simulink model "simulink_mecha"  (R2016b)
settings: Solver=VariableStepAuto  StartTime=0.0  StopTime=50  RelTol=1e-3
libraries: aerolibutil x1, simulink x1
settings Model: Creator=Utente  LastModifiedBy=liana

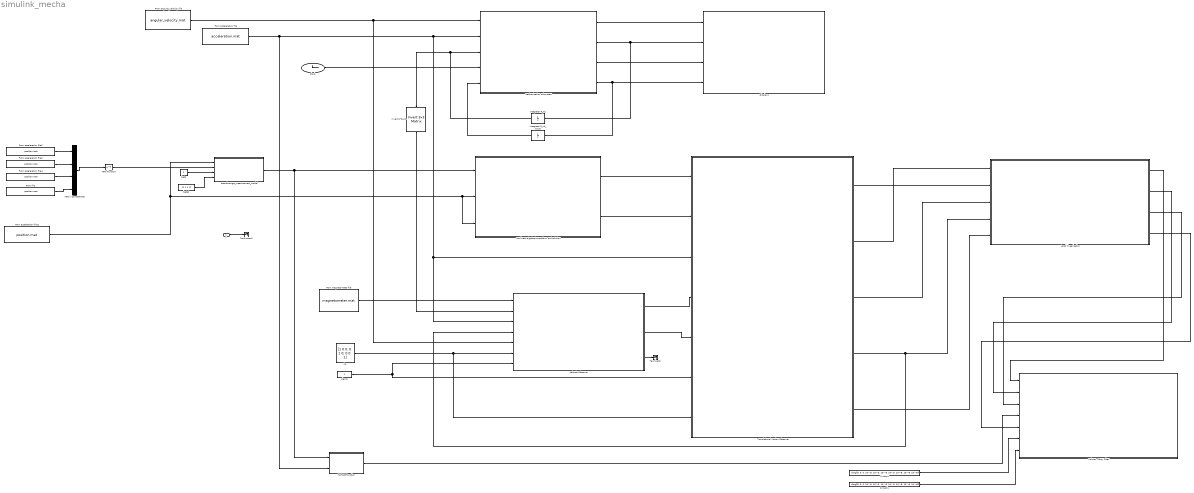
== system simulink_mecha ==
  f : Inport
  Attitude Observer : Subsystem
  Clock : Clock
  Displays : Subsystem
  From acceleration file : FromFile  FileName=acceleration.mat  SampleTime=0
  From acceleration file{1..4} (4 alike) : FromFile  FileName=position.mat  SampleTime=0
  From angular_velocity file : FromFile  FileName=angular_velocity.mat  SampleTime=0
  From file : FromFile  FileName=position.mat  SampleTime=0
  From magnetometer file : FromFile  FileName=magnetometer.mat  SampleTime=0  InterpolationWithinTimeRange=Zero order hold
  Integrator R_nb : Integrator
  Integrator R_nb_noise : Integrator
  Invert of R_nb : aerolibutil/Invert  3x3 Matrix
  Kalman - Bucy Filter : Subsystem
  Kp : Constant  Value=[1 0 0; 0 1 0; 0 0 1]
  Local linearization : Subsystem
  MATLAB Function : MATLAB Function  TreatAsAtomicUnit=on
  Math Function : Math  Operator=transpose  SaturateOnIntegerOverflow=on
  Matrix Concatenate : Concatenate  NumInputs=4  Mode=Multidimensional array  ConcatenateDimension=2
  Mechanisation subsystem : Subsystem
  Nonlinear algebraic transform and solution : Subsystem
  Q matrix : Constant  Value=diag([0, 0, 0, 10^-5, 10^-3, 10^-3, 10^-3, 10^-8, 10^-8, 10^-8])
  R matrix : Constant  Value=diag([0, 0, 0, 10^-5, 10^-3, 10^-3, 10^-3, 10^-8, 10^-8, 10^-8])
  Terminator : Terminator
  Terminator1 : Terminator
  Translational Motion Observer : Subsystem
  beta : Constant
  beta1 : Constant  Value=[1 1 1 1]
  pseudorange_measurement_model : MATLAB Function  TreatAsAtomicUnit=on
  sigma : Constant
  wires:
  From angular_velocity file/1 -> Attitude Observer/5(w_ib), Mechanisation subsystem/1(w_ib)
  Clock/1 -> Mechanisation subsystem/4(t)
  Mechanisation subsystem/2(R_nb_dot) -> Integrator R_nb/1, Displays/2(R_nb_dot)
  Integrator R_nb/1 -> Invert of R_nb/1, Mechanisation subsystem/3(R_nb)
  Mechanisation subsystem/1(v_n_dot) -> Displays/1(v_n_dot)
  Mechanisation subsystem/3(v_n_dot_noise) -> Displays/3(v_n_dot_noise)
  Mechanisation subsystem/4(R_nb_dot_noise) -> Integrator R_nb_noise/1, Displays/4(R_nb_dot_noise)
  Integrator R_nb_noise/1 -> Mechanisation subsystem/5(R_nb_noise)
  Invert of R_nb/1 -> Attitude Observer/2(R_bn)
  From magnetometer file/1 -> Attitude Observer/1(m_b_mag)
  Nonlinear algebraic transform and solution/1(delta) -> Translational Motion Observer/1(delta)
  Translational Motion Observer/4(f_n_stim) -> Local linearization/4(f_n_stim), Attitude Observer/4(f_n_stim)
  Attitude Observer/1(J) -> Translational Motion Observer/4(J)
  Attitude Observer/2(R_nb_stim) -> Translational Motion Observer/5(R_nb_stim)
  Attitude Observer/3(b_stim) -> Terminator/1
  From acceleration file1/1 -> pseudorange_measurement_model/1(p_n), Nonlinear algebraic transform and solution/3(p0), Nonlinear algebraic transform and solution/2(p)
  Kp/1 -> Translational Motion Observer/7(Kp), Attitude Observer/6(Kp)
  sigma/1 -> Translational Motion Observer/6(sigma), Attitude Observer/7(sigma)
  Translational Motion Observer/2(p_n_stim) -> Local linearization/1(p_n_stim)
  Translational Motion Observer/3(v_n_stim) -> Local linearization/3(v_n_stim)
  Nonlinear algebraic transform and solution/2(C_dx) -> Translational Motion Observer/2(C_dx)
  Translational Motion Observer/5(system) -> Local linearization/5(system)
  Translational Motion Observer/1(beta_stim) -> Local linearization/2(beta_stim)
  Local linearization/1(AL) -> Kalman - Bucy Filter/1(AL)
  Local linearization/2(BL) -> Kalman - Bucy Filter/2(BL)
  Local linearization/3(CL) -> Kalman - Bucy Filter/3(CL)
  MATLAB Function/1(z_k) -> Kalman - Bucy Filter/4(sensors measurements)
  From acceleration file/1 -> MATLAB Function/2(f_n), Attitude Observer/3(f_b), Translational Motion Observer/3(f_b_imu), Mechanisation subsystem/2(f_b)
  pseudorange_measurement_model/1(y) -> MATLAB Function/1(range), Nonlinear algebraic transform and solution/1(y)
  Local linearization/4(U) -> Kalman - Bucy Filter/5(U)
  f/1 -> Terminator1/1
  beta/1 -> pseudorange_measurement_model/3(beta)
  beta1/1 -> pseudorange_measurement_model/4(epsilon)
  From acceleration file2/1 -> Matrix Concatenate/1
  From acceleration file3/1 -> Matrix Concatenate/2
  From acceleration file4/1 -> Matrix Concatenate/3
  From file/1 -> Matrix Concatenate/4
  Matrix Concatenate/1 -> Math Function/1
  Math Function/1 -> pseudorange_measurement_model/2(p_n_i)
  R matrix/1 -> Kalman - Bucy Filter/6(R)
  Q matrix/1 -> Kalman - Bucy Filter/7(Q)

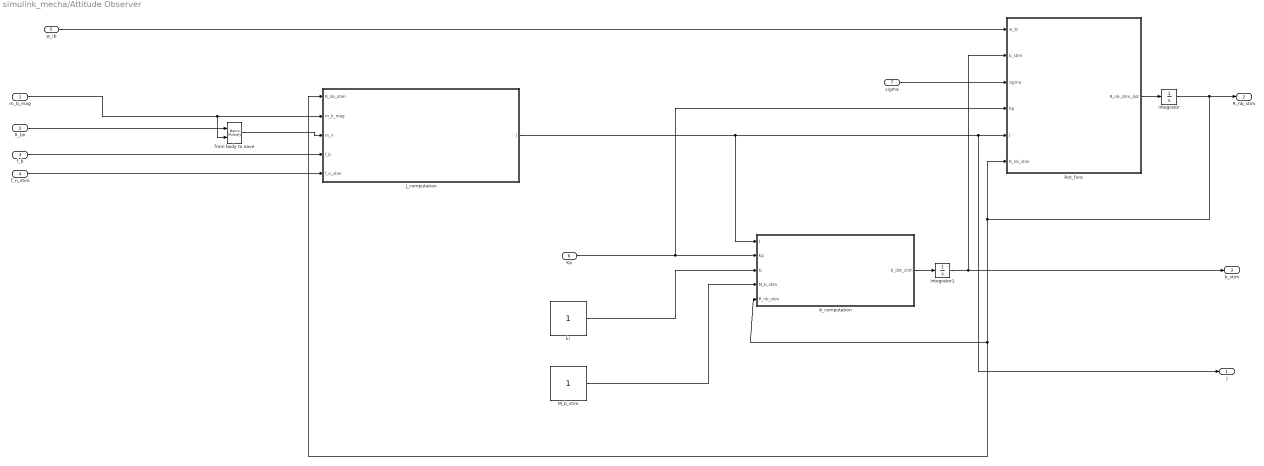
== system simulink_mecha/Attitude Observer ==
  m_b_mag : Inport
  R_bn : Inport  Port=2
  f_b : Inport  Port=3
  f_n_stim : Inport  Port=4
  w_ib : Inport  Port=5
  Kp : Inport  Port=6
  sigma : Inport  Port=7
  Integrator : Integrator
  Integrator1 : Integrator
  J_computation : Subsystem
  M_b_stim : Constant
  Rot_func : MATLAB Function  TreatAsAtomicUnit=on
  b_computation : MATLAB Function  TreatAsAtomicUnit=on
  from body to nave : Product  Multiplication=Matrix(*)
  ki : Constant
  J : Outport
  R_nb_stim : Outport  Port=2
  b_stim : Outport  Port=3
  wires:
  m_b_mag/1 -> from body to nave/2, J_computation/2(m_b_mag)
  Rot_func/1(R_nb_stim_dot) -> Integrator/1
  b_computation/1(b_dot_stim) -> Integrator1/1
  Integrator/1 -> J_computation/1(R_nb_stim), b_computation/5(R_nb_stim), Rot_func/6(R_nb_stim), R_nb_stim/1
  Integrator1/1 -> b_stim/1, Rot_func/2(b_stim)
  from body to nave/1 -> J_computation/3(m_n)
  f_b/1 -> J_computation/4(f_b)
  f_n_stim/1 -> J_computation/5(f_n_stim)
  J_computation/1(J) -> b_computation/1(J), J/1, Rot_func/5(J)
  Kp/1 -> Rot_func/4(Kp), b_computation/2(Kp)
  ki/1 -> b_computation/3(ki)
  M_b_stim/1 -> b_computation/4(M_b_stim)
  sigma/1 -> Rot_func/3(sigma)
  w_ib/1 -> Rot_func/1(w_ib)
  R_bn/1 -> from body to nave/1

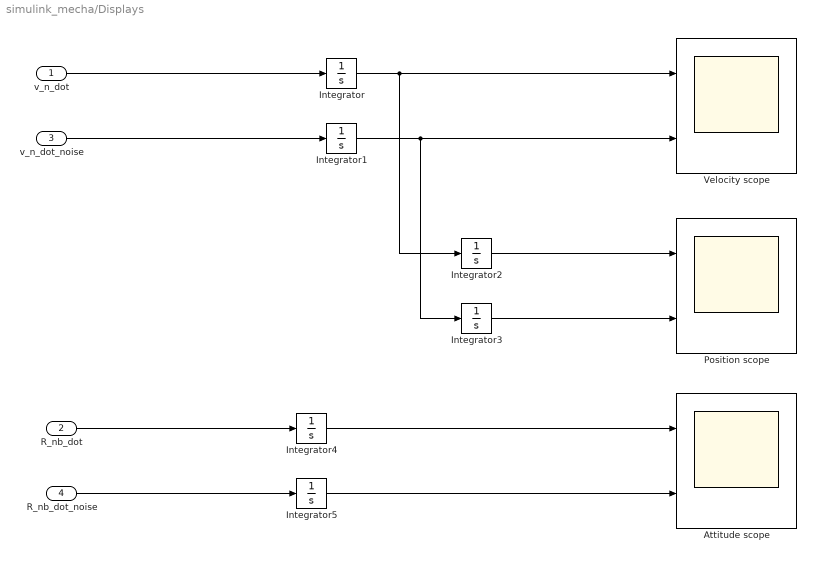
== system simulink_mecha/Displays ==
  v_n_dot : Inport
  R_nb_dot : Inport  Port=2
  v_n_dot_noise : Inport  Port=3
  R_nb_dot_noise : Inport  Port=4
  Attitude scope : Scope  NumInputPorts=2
  Integrator{,1..5} (6 alike) : Integrator
  Position scope : Scope  NumInputPorts=2
  Velocity scope : Scope  NumInputPorts=2
  wires:
  v_n_dot/1 -> Integrator/1
  v_n_dot_noise/1 -> Integrator1/1
  Integrator/1 -> Integrator2/1, Velocity scope/1
  Integrator1/1 -> Integrator3/1, Velocity scope/2
  Integrator2/1 -> Position scope/1
  Integrator3/1 -> Position scope/2
  R_nb_dot/1 -> Integrator4/1
  R_nb_dot_noise/1 -> Integrator5/1
  Integrator4/1 -> Attitude scope/1
  Integrator5/1 -> Attitude scope/2

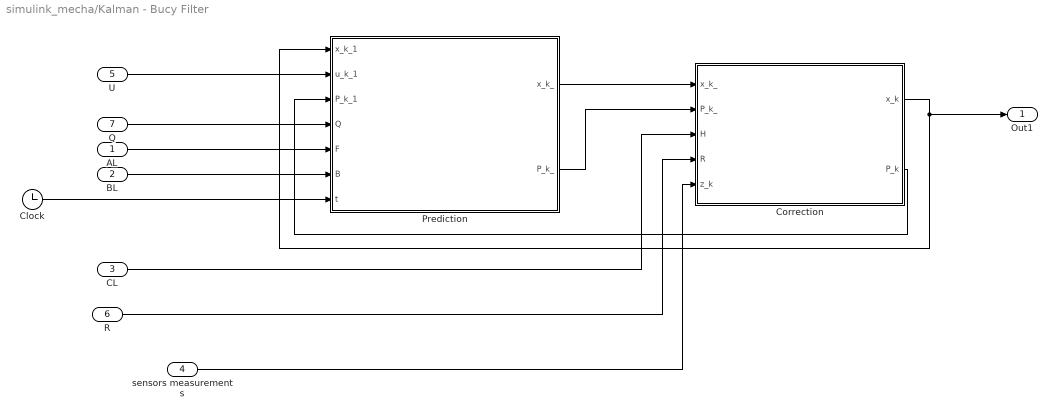
== system simulink_mecha/Kalman - Bucy Filter ==
  AL : Inport
  BL : Inport  Port=2
  CL : Inport  Port=3
  sensors measurements : Inport  Port=4
  U : Inport  Port=5
  R : Inport  Port=6
  Q : Inport  Port=7
  Clock : Clock
  Correction : MATLAB Function  TreatAsAtomicUnit=on
  Prediction : MATLAB Function  TreatAsAtomicUnit=on
  Out1 : Outport
  wires:
  Prediction/2(P_k_) -> Correction/2(P_k_)
  Prediction/1(x_k_) -> Correction/1(x_k_)
  Correction/2(P_k) -> Prediction/3(P_k_1)
  Correction/1(x_k) -> Prediction/1(x_k_1), Out1/1
  AL/1 -> Prediction/5(F)
  CL/1 -> Correction/3(H)
  Clock/1 -> Prediction/7(t)
  Q/1 -> Prediction/4(Q)
  sensors measurements/1 -> Correction/5(z_k)
  BL/1 -> Prediction/6(B)
  U/1 -> Prediction/2(u_k_1)
  R/1 -> Correction/4(R)

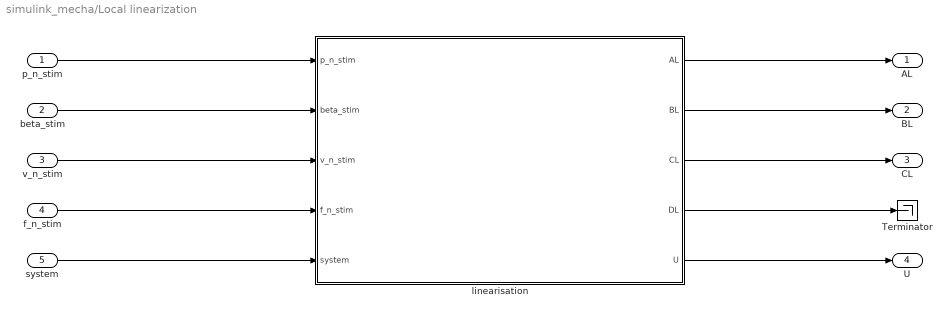
== system simulink_mecha/Local linearization ==
  p_n_stim : Inport
  beta_stim : Inport  Port=2
  v_n_stim : Inport  Port=3
  f_n_stim : Inport  Port=4
  system : Inport  Port=5
  Terminator : Terminator
  linearisation : MATLAB Function  TreatAsAtomicUnit=on
  AL : Outport
  BL : Outport  Port=2
  CL : Outport  Port=3
  U : Outport  Port=4
  wires:
  system/1 -> linearisation/5(system)
  p_n_stim/1 -> linearisation/1(p_n_stim)
  beta_stim/1 -> linearisation/2(beta_stim)
  v_n_stim/1 -> linearisation/3(v_n_stim)
  f_n_stim/1 -> linearisation/4(f_n_stim)
  linearisation/1(AL) -> AL/1
  linearisation/2(BL) -> BL/1
  linearisation/3(CL) -> CL/1
  linearisation/4(DL) -> Terminator/1
  linearisation/5(U) -> U/1

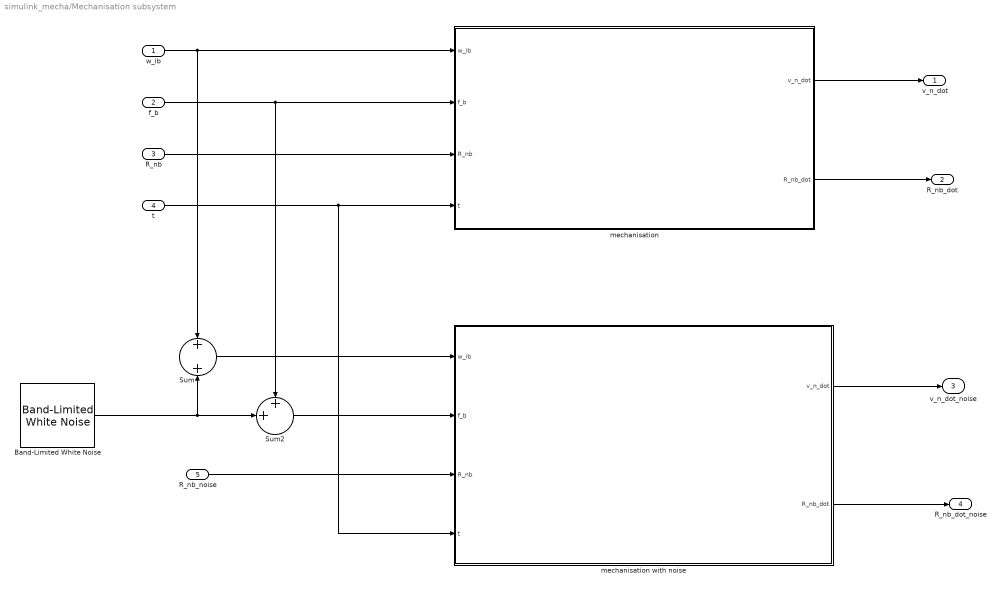
== system simulink_mecha/Mechanisation subsystem ==
  w_ib : Inport
  f_b : Inport  Port=2
  R_nb : Inport  Port=3
  t : Inport  Port=4
  R_nb_noise : Inport  Port=5
  Band-Limited White Noise : simulink/Sources/Band-Limited White Noise  Cov=[100 100 100]'  Ts=0.1  seed=[23341]  VectorParams1D=off
  Sum : Sum  Inputs=+|+
  Sum2 : Sum  Inputs=++|
  mechanisation : MATLAB Function  TreatAsAtomicUnit=on
  mechanisation with noise : MATLAB Function  TreatAsAtomicUnit=on
  v_n_dot : Outport
  R_nb_dot : Outport  Port=2
  v_n_dot_noise : Outport  Port=3
  R_nb_dot_noise : Outport  Port=4
  wires:
  w_ib/1 -> mechanisation/1(w_ib), Sum/1
  t/1 -> mechanisation with noise/4(t), mechanisation/4(t)
  R_nb/1 -> mechanisation/3(R_nb)
  f_b/1 -> Sum2/1, mechanisation/2(f_b)
  mechanisation/1(v_n_dot) -> v_n_dot/1
  mechanisation/2(R_nb_dot) -> R_nb_dot/1
  Band-Limited White Noise/1 -> Sum/2, Sum2/2
  Sum/1 -> mechanisation with noise/1(w_ib)
  Sum2/1 -> mechanisation with noise/2(f_b)
  mechanisation with noise/1(v_n_dot) -> v_n_dot_noise/1
  mechanisation with noise/2(R_nb_dot) -> R_nb_dot_noise/1
  R_nb_noise/1 -> mechanisation with noise/3(R_nb)

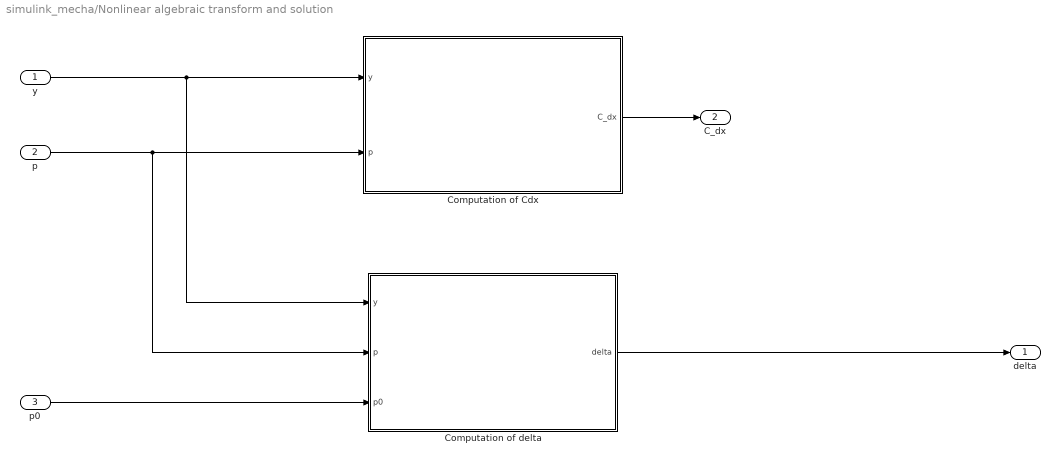
== system simulink_mecha/Nonlinear algebraic transform and solution ==
  y : Inport
  p : Inport  Port=2
  p0 : Inport  Port=3
  Computation of Cdx : MATLAB Function  TreatAsAtomicUnit=on
  Computation of delta : MATLAB Function  TreatAsAtomicUnit=on
  delta : Outport
  C_dx : Outport  Port=2
  wires:
  y/1 -> Computation of delta/1(y), Computation of Cdx/1(y)
  p/1 -> Computation of delta/2(p), Computation of Cdx/2(p)
  p0/1 -> Computation of delta/3(p0)
  Computation of delta/1(delta) -> delta/1
  Computation of Cdx/1(C_dx) -> C_dx/1

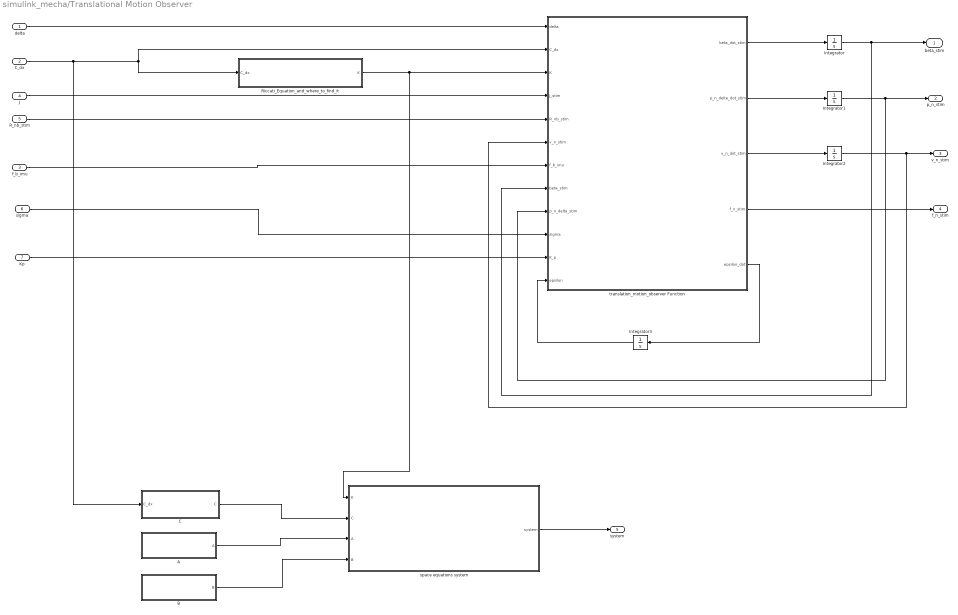
== system simulink_mecha/Translational Motion Observer ==
  delta : Inport
  C_dx : Inport  Port=2
  f_b_imu : Inport  Port=3
  J : Inport  Port=4
  R_nb_stim : Inport  Port=5
  sigma : Inport  Port=6
  Kp : Inport  Port=7
  A : MATLAB Function  TreatAsAtomicUnit=on
  B : MATLAB Function  TreatAsAtomicUnit=on
  C : MATLAB Function  TreatAsAtomicUnit=on
  Integrator{,1..3} (4 alike) : Integrator
  Riccati_Equation_and_where_to_find_it : Subsystem
  space equations system : MATLAB Function  TreatAsAtomicUnit=on
  translation_motion_observer Function : MATLAB Function  TreatAsAtomicUnit=on
  beta_stim : Outport
  p_n_stim : Outport  Port=2
  v_n_stim : Outport  Port=3
  f_n_stim : Outport  Port=4
  system : Outport  Port=5
  wires:
  translation_motion_observer Function/4(f_n_stim) -> f_n_stim/1
  translation_motion_observer Function/3(v_n_dot_stim) -> Integrator2/1
  Integrator2/1 -> translation_motion_observer Function/6(v_n_stim), v_n_stim/1
  translation_motion_observer Function/2(p_n_delta_dot_stim) -> Integrator1/1
  Integrator1/1 -> translation_motion_observer Function/9(p_n_delta_stim), p_n_stim/1
  Integrator/1 -> translation_motion_observer Function/8(beta_stim), beta_stim/1
  translation_motion_observer Function/1(beta_dot_stim) -> Integrator/1
  translation_motion_observer Function/5(epsilon_dot) -> Integrator3/1
  Integrator3/1 -> translation_motion_observer Function/12(epsilon)
  C_dx/1 -> C/1(C_dx), translation_motion_observer Function/2(C_dx), Riccati_Equation_and_where_to_find_it/1(C_dx)
  J/1 -> translation_motion_observer Function/4(J_stim)
  R_nb_stim/1 -> translation_motion_observer Function/5(R_nb_stim)
  delta/1 -> translation_motion_observer Function/1(delta)
  f_b_imu/1 -> translation_motion_observer Function/7(f_b_imu)
  sigma/1 -> translation_motion_observer Function/10(sigma)
  Kp/1 -> translation_motion_observer Function/11(K_p)
  A/1(A) -> space equations system/3(A)
  C/1(C) -> space equations system/2(C)
  Riccati_Equation_and_where_to_find_it/1(K) -> space equations system/1(K), translation_motion_observer Function/3(K)
  B/1(B) -> space equations system/4(B)
  space equations system/1(system) -> system/1

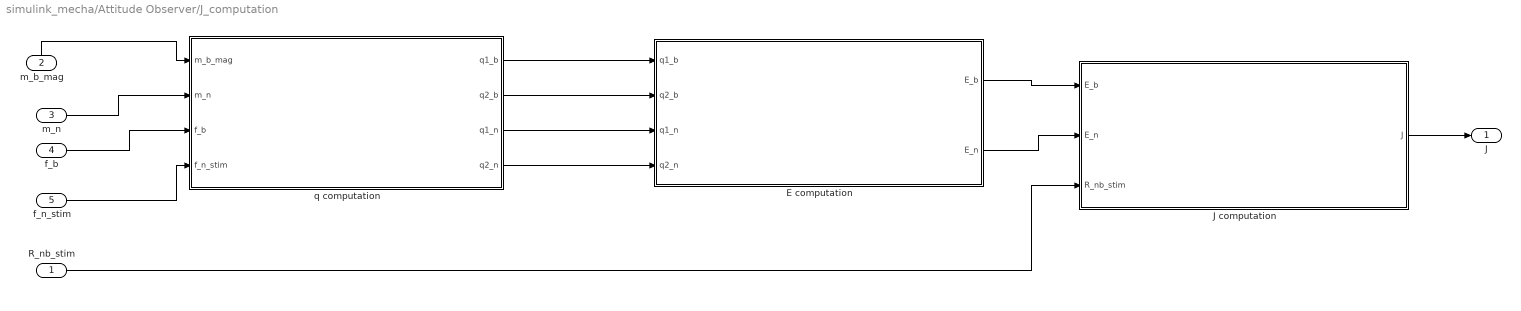
== system simulink_mecha/Attitude Observer/J_computation ==
  R_nb_stim : Inport
  m_b_mag : Inport  Port=2
  m_n : Inport  Port=3
  f_b : Inport  Port=4
  f_n_stim : Inport  Port=5
  E computation : MATLAB Function  TreatAsAtomicUnit=on
  J computation : MATLAB Function  TreatAsAtomicUnit=on
  q computation : MATLAB Function  TreatAsAtomicUnit=on
  J : Outport
  wires:
  E computation/2(E_n) -> J computation/2(E_n)
  E computation/1(E_b) -> J computation/1(E_b)
  q computation/4(q2_n) -> E computation/4(q2_n)
  q computation/3(q1_n) -> E computation/3(q1_n)
  q computation/1(q1_b) -> E computation/1(q1_b)
  m_n/1 -> q computation/2(m_n)
  J computation/1(J) -> J/1
  R_nb_stim/1 -> J computation/3(R_nb_stim)
  f_n_stim/1 -> q computation/4(f_n_stim)
  m_b_mag/1 -> q computation/1(m_b_mag)
  q computation/2(q2_b) -> E computation/2(q2_b)
  f_b/1 -> q computation/3(f_b)

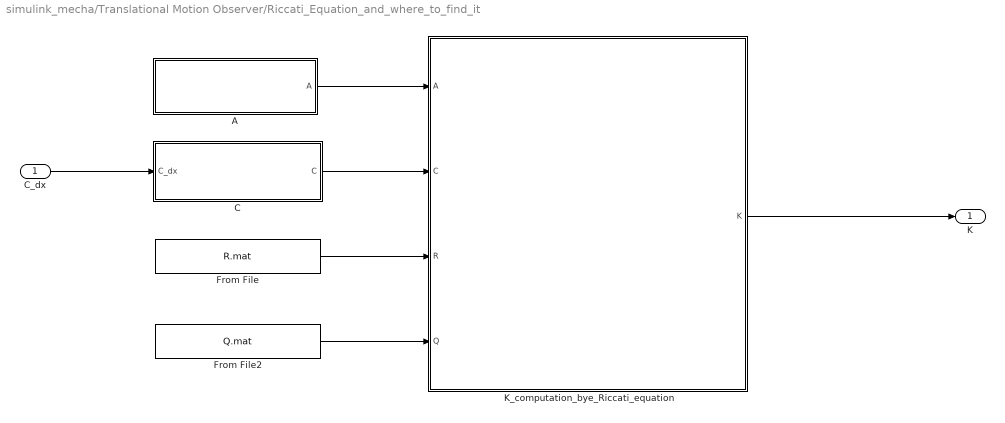
== system simulink_mecha/Translational Motion Observer/Riccati_Equation_and_where_to_find_it ==
  C_dx : Inport
  A : MATLAB Function  TreatAsAtomicUnit=on
  C : MATLAB Function  TreatAsAtomicUnit=on
  From File : FromFile  FileName=R.mat  SampleTime=0
  From File2 : FromFile  FileName=Q.mat  SampleTime=0
  K_computation_bye_Riccati_equation : MATLAB Function  TreatAsAtomicUnit=on
  K : Outport
  wires:
  C_dx/1 -> C/1(C_dx)
  K_computation_bye_Riccati_equation/1(K) -> K/1
  From File/1 -> K_computation_bye_Riccati_equation/3(R)
  A/1(A) -> K_computation_bye_Riccati_equation/1(A)
  From File2/1 -> K_computation_bye_Riccati_equation/4(Q)
  C/1(C) -> K_computation_bye_Riccati_equation/2(C)

== matlab function simulink_mecha/Attitude Observer/J_computation/E computation ==
  data: q1_b input; E_b output; q2_b input; q1_n input; q2_n input; E_n output
function [E_b, E_n]= Efunc(q1_b, q2_b, q1_n, q2_n)



E_b = (q1_b, skew(q1_b)*q2_b, (skew(q1_b)*skew(q1_b))*q2_b);
E_n = (q1_n, skew(q1_n)*q2_n, (skew(q1_n)*skew(q1_n))*q2_n);

== matlab function simulink_mecha/Attitude Observer/J_computation/q computation ==
  data: m_b_mag input; q1_b output; m_n input; f_b input; f_n_stim input; q2_b output; q1_n output; q2_n output
function [q1_b, q2_b, q1_n, q2_n] = qfunc(m_b_mag, m_n, f_b, f_n_stim)

g_n = [0 0 1]';

q1_b = m_b_mag/norm(m_b_mag,2);
q2_b = f_b/norm(g_n,2);

q1_n = m_n/norm(m_n,2);
q2_n = f_n_stim/norm(g_n,2);

== matlab function simulink_mecha/Kalman - Bucy Filter/Prediction ==
  data: x_k_1 input; x_k_ output; u_k_1 input; P_k_1 input; Q input; F input; B input; P_k_ output; t input
function [x_k_, P_k_] = prediction(x_k_1, u_k_1, P_k_1, Q, F,B, t)

    % initial value of x_k_1
    if t == 0
        x_k_1 = zeros(10,1);
    end

    x_k_ = F * x_k_1 + B * u_k_1;
    
    P_k_ = F * P_k_1 * F' + Q;
    

end

== matlab function simulink_mecha/Mechanisation subsystem/mechanisation ==
  data: w_ib input; f_b input; v_n_dot output; R_nb_dot output; R_nb input; t input
function [v_n_dot, R_nb_dot] = mechanisation(w_ib, f_b, R_nb, t)



g_n = [0 0 1]';

% w_ib = size(3,1);

if t == 0
    v_n_dot = zeros(3,1);
    R_nb_dot = zeros(3,3);
    R_nb = eye(3);
end

% mechanisation

% Skew = zeros(3,3);
% Skew(1,2) = -w_ib(3);
% Skew(2,1) = w_ib(3);
% Skew(1,3) = w_ib(2);
% Skew(3,1) = -w_ib(2);
% Skew(2,3) = -w_ib(1);
% Skew(3,2) = w_ib(1);

Skew = skew(w_ib);


%p_dot = v_n;
v_n_dot = R_nb * f_b + g_n;
R_nb_dot = R_nb * Skew;

== matlab function simulink_mecha/Mechanisation subsystem/mechanisation with noise ==
  data: w_ib input; f_b input; v_n_dot output; R_nb_dot output; R_nb input; t input
function [v_n_dot, R_nb_dot] = mechanisation(w_ib, f_b, R_nb, t)



g_n = [0 0 1]';

% w_ib = size(3,1);

if t == 0
    v_n_dot = zeros(3,1);
    R_nb_dot = zeros(3,3);
    R_nb = eye(3);
end

% mechanisation

% Skew = zeros(3,3);
% Skew(1,2) = -w_ib(3);
% Skew(2,1) = w_ib(3);
% Skew(1,3) = w_ib(2);
% Skew(3,1) = -w_ib(2);
% Skew(2,3) = -w_ib(1);
% Skew(3,2) = w_ib(1);
Skew = skew(w_ib);


%p_dot = v_n;
v_n_dot = R_nb * f_b + g_n;
R_nb_dot = R_nb * Skew;

== matlab function simulink_mecha/Attitude Observer/J_computation/J computation ==
  data: E_b input; J output; E_n input; R_nb_stim input
function J = Jfunc(E_b, E_n, R_nb_stim)


J = (E_n - R_nb_stim * E_b) * (E_b');

== matlab function simulink_mecha/Attitude Observer/b_computation ==
  data: J input; b_dot_stim output; Kp input; ki input; M_b_stim input; R_nb_stim input
function b_dot_stim = b_dot_stim_func(J, Kp, ki, M_b_stim, R_nb_stim)

% don't break balls if there are too rows

SAT = sat(R_nb_stim)';
PA = Pa( SAT * Kp * J);
VEX = vexfunc(PA);
b_dot_stim = Proj( -ki * VEX, M_b_stim);

== matlab function simulink_mecha/Translational Motion Observer/translation_motion_observer Function ==
  data: delta input; C_dx input; K input; beta_dot_stim output; J_stim input; R_nb_stim input; p_n_delta_dot_stim output; v_n_dot_stim output; f_n_stim output; v_n_stim input; f_b_imu input; beta_stim input; p_n_delta_stim input; sigma input; K_p input; epsilon_dot output; epsilon input
function [beta_dot_stim,p_n_delta_dot_stim,v_n_dot_stim,f_n_stim,epsilon_dot] =  TMO_func(delta,C_dx,K,J_stim,R_nb_stim, v_n_stim,f_b_imu, beta_stim, p_n_delta_stim,sigma,K_p,epsilon)

 K_pp = K(1:3,:); 
 K_beta_p = K(4,:);
 K_v_p = K(5:7,:);
 K_eps_p = K(8:10,:);
 %obtained by Riccati equation..


% remember to insert a clock to define dimensions of all variables

g_n = [0 0 1]';

x_stim = [p_n_delta_stim beta_stim];
delta_stim = 2*C_dx*x_stim;
delta_diff = (delta - delta_stim);



p_n_delta_dot_stim = v_n_stim + K_pp * delta_diff;        % eq 14


beta_dot_stim = K_beta_p * delta_diff;                       % eq 15


%theoretically we can't know epsilon
f_n_stim = R_nb_stim*f_b_imu + epsilon ;         % eq 18


v_n_dot_stim  = f_n_stim + g_n + K_v_p*delta_diff;         % eq 16


epsilon_dot   = -sigma*K_p*J_stim*f_b_imu + K_eps_p*delta_diff; % eq 17
end

== matlab function simulink_mecha/Nonlinear algebraic transform and solution/Computation of Cdx ==
  data: y input; p input; C_dx output
function C_dx  = C_dx_func(y,p)

    % y vector 
    % p matrix has row vectors
    %            (x,y,z) cols 
    %            m-rows are the numbers of the transponders
    % all variables are in navigation frame oh yeah! baby ;)
    
    [row,col] = size(p);
    [row_,col_] = size(y);
    
    % m-measure vector
    p_m = p(row,:);
    y_m = y(row_);

    
    p_ = [];
    y_ = [];
    
    for i = 1 : 1 : row-1
    
        p_ = [p_ ; p_m - p(i,:)];
        y_ = [y_ ; y(i) - y_m];
        
    end
    
    C_dx = [p_ y_];

end

== matlab function simulink_mecha/Nonlinear algebraic transform and solution/Computation of delta ==
  data: y input; delta output size=3; p input; p0 input
function delta  = delta_func(y,p,p0)

    % y vector 
    % p matrix has row vectors
    %            (x,y,z) cols 
    %            m-rows are the numbers of the transponders
    % all variables are in navigation frame oh yeah! baby ;)
    % z is a col vector of scalars
    
    % we must choose p0 (a block)
    
    [row,col] = size(p);
    %[row_,col_] = size(y);
    
    p_los = [ ];
    z = [ ];
    %defining los vector
    
    for i = 1:1:row-1
       N = p(i,:) - p0;
       p_los = [p_los N]; 
       %p_los(i,:) = p(i,:) - p0;
    end
    
    p_los = p_los';
    
    for i = 1:1:row-1
        z= [z y(i)^2-norm(p_los(i,:))^2];
    end
    
    z = z';
    
    delta = [];
    
    for i = 1:1:row-1
        delta = [delta z(i) - z_m] ; %amm fenito
    end
    
    delta = delta';

end

== matlab function simulink_mecha/Translational Motion Observer/Riccati_Equation_and_where_to_find_it/K_computation_bye_Riccati_equation ==
  data: A input; K output; C input; R input; Q input
function K = K_func(A,C,R,Q)

K = zeros(10,10);

coder.extrinsic('care');

[P,L,G] = care(A,C',Q,R);

R_inv = pinv(R); 

K = P*C'*R_inv;

== matlab function simulink_mecha/Translational Motion Observer/Riccati_Equation_and_where_to_find_it/A ==
  data: A output
function A = A()

 A = zeros(10);

 A(1:3,5:7) = eye(3);
 A(5:7,8:10) = eye(3);
 
A;

== matlab function simulink_mecha/Translational Motion Observer/Riccati_Equation_and_where_to_find_it/C ==
  data: C output; C_dx input
function C = C(C_dx)

   row = size(C_dx,1); 

   C1 = zeros(row,6);

 C = [2*C_dx C1];

== matlab function simulink_mecha/Attitude Observer/Rot_func ==
  data: R_nb_stim_dot output; w_ib input; b_stim input; sigma input; Kp input; J input; R_nb_stim input
function R_nb_stim_dot = rot_func(w_ib,b_stim,sigma,Kp,J,R_nb_stim) 

Skew = skew(w_ib - b_stim);

R_nb_stim_dot = R_nb_stim * Skew + sigma * Kp * J;

== matlab function simulink_mecha/Kalman - Bucy Filter/Correction ==
  data: x_k_ input; P_k_ input; H input; R input; z_k input; x_k output; P_k output
function [x_k, P_k] = correction(x_k_ ,P_k_, H, R, z_k)

    n = size(P_k_);


    K_k = P_k_ * H' * pinv(H * P_k_ * H' + R);
    
    x_k = x_k_ + K_k * (z_k - H * x_k_);
    
    P_k = (eye(n) - K_k * H)*P_k_;

end

== matlab function simulink_mecha/MATLAB Function ==
  data: range input; f_n input; z_k output
function z_k = fcn(range,f_n)

% dirty values for kalman

z_k = [f_n; range];

== matlab function simulink_mecha/Translational Motion Observer/space equations system ==
  data: K input; system output; C input; A input; B input
function system = build_sys(K, C, A, B)

system = sys(A-K*C,B,C,0);

end

== matlab function simulink_mecha/Translational Motion Observer/A ==
  data: A output
function A = A()

 A = zeros(10);

 A(1:3,5:7) = eye(3);
 A(5:7,8:10) = eye(3);
 
end

== matlab function simulink_mecha/Translational Motion Observer/C ==
  data: C output; C_dx input
function C = C(C_dx)

   row = size(C_dx,1); 

   C1 = zeros(row,6);

 C = [2*C_dx C1];
 
 
end

== matlab function simulink_mecha/Translational Motion Observer/B ==
  data: B output
function B = B()

 B = zeros(10,3);

 B(8:10,1:3) = eye(3);
end

== matlab function simulink_mecha/Local linearization/linearisation ==
  data: p_n_stim input; beta_stim input; v_n_stim input; f_n_stim input; system input; AL output; BL output; CL output; DL output; U output
function [AL, BL, CL, DL, U] = linearisation(p_n_stim,beta_stim, v_n_stim, f_n_stim, system)

 % building state vector
  xsi = zeros(10,1);
  xsi(1:3,1) = p_n_stim;
  xsi(4,1) = beta_stim;
  xsi(5:7,1) = v_n_stim;
  xsi(8:10,1) = f_n_stim;
  
  
  % xsi = [p_n_stim ; beta_stim; v_n_stim; f_n_tim];

% getting work point

[X,U,Y,DX] = trim('system', xsi);

% computing linearisation model

[AL, BL, CL, DL] = linmod('system',X,U);

end

== matlab function simulink_mecha/pseudorange_measurement_model ==
  data: p_n input; y output size=4; p_n_i input; beta input; epsilon input
function y = pseudorange_mea_model(p_n,p_n_i,beta,epsilon)

  %  row-vector


  y = [];

  for i = 1: size(p_n_i,1)

      rho = norm(p_n-p_n_i(i,:));  % eq. 7
      
      y_ = rho + beta + epsilon(i); % eq. 8
      
      y = [y, y_];  

  end
      
y;
